simulink model "dc_motor_control"  (R2025b)
settings: Solver=VariableStepAuto  StartTime=0.0  StopTime=60  RelTol=1e-3
undefined symbols (not defined in the file): b, J, Ke, Kt, L, R
settings Model: Creator=ENG. Hussein Issa  LastModifiedBy=ENG. Hussein Issa

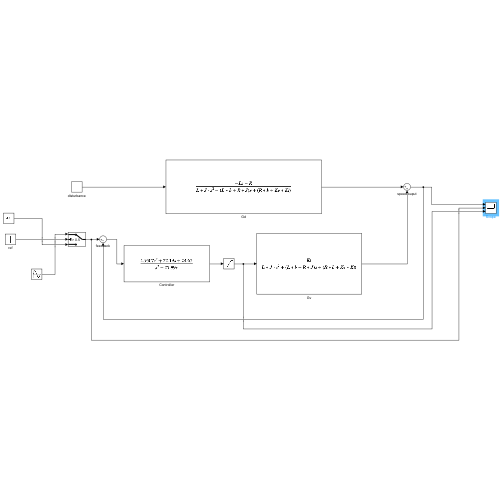
[thumbnail: Simulink's stored preview of the top-level diagram]
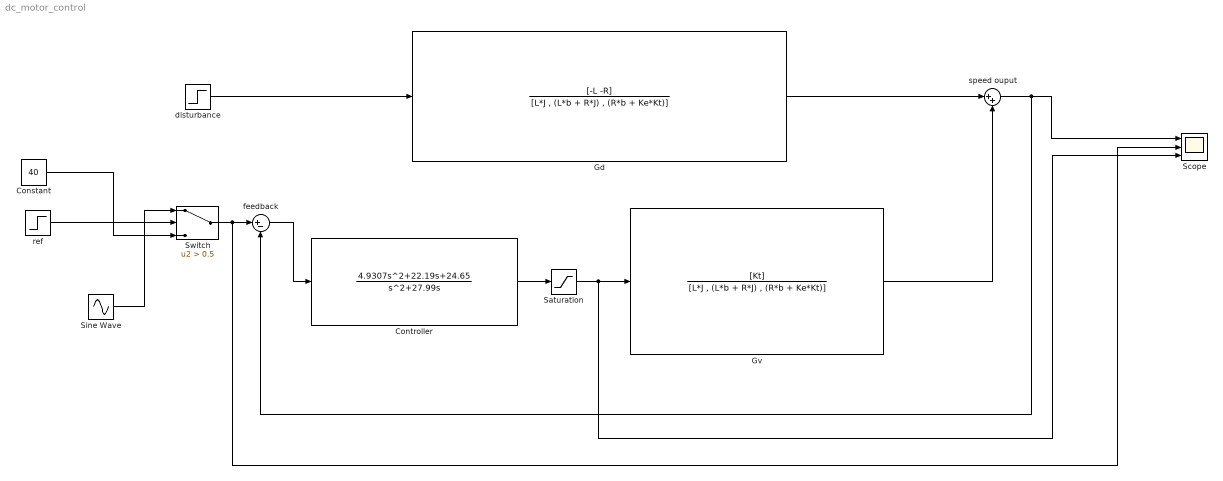
== system dc_motor_control ==
  Constant : Constant  Value=40
  Controller : TransferFcn  Numerator=[4.9307 22.19 24.65]  Denominator=[1 27.99 0]
  Gd : TransferFcn  Numerator=[-L -R]  Denominator=[L*J , (L*b + R*J) , (R*b + Ke*Kt)]
  Gv : TransferFcn  Numerator=[Kt]  Denominator=[L*J , (L*b + R*J) , (R*b + Ke*Kt)]
  Saturation : Saturate  UpperLimit=12  LowerLimit=-12
  Scope : Scope  NumInputPorts=3
      settings: ActiveDisplayYMinimum=-19.834959133678787  ActiveDisplayYMaximum=58.5146322031091
  Sine Wave : Sin  Amplitude=5  Bias=40  Frequency=0.5  SampleTime=0
  Switch : Switch  Criteria=u2 > Threshold  Threshold=0.5  SaturateOnIntegerOverflow=off  InputSameDT=off
  disturbance : Step  Time=20  After=0  SampleTime=0
  feedback : Sum  Inputs=|+-
  ref : Step  Time=10  SampleTime=0
  speed ouput : Sum  Inputs=|++
  wires:
  disturbance/1 -> Gd/1
  feedback/1 -> Controller/1
  Gd/1 -> speed ouput/1
  Gv/1 -> speed ouput/2
  speed ouput/1 -> feedback/2, Scope/1
  Controller/1 -> Saturation/1
  Saturation/1 -> Gv/1, Scope/3
  Switch/1 -> Scope/2, feedback/1
  ref/1 -> Switch/2
  Constant/1 -> Switch/3
  Sine Wave/1 -> Switch/1
